simulink model "wptv1"  (R2024b)
settings: Solver=ode23tb  StartTime=0.0  StopTime=0.05  MaxStep=1e-7  RelTol=1e-3
libraries: spsSeriesRLCBranchLib x7, spsDiodeLib x5, spsMosfetLib x5, spsVoltageMeasurementLib x3, spsDCVoltageSourceLib x1, spsGroundLib x1, spsMutualInductanceLib x1, sps_lib x1
settings Model: Creator=barad  LastModifiedBy=barad

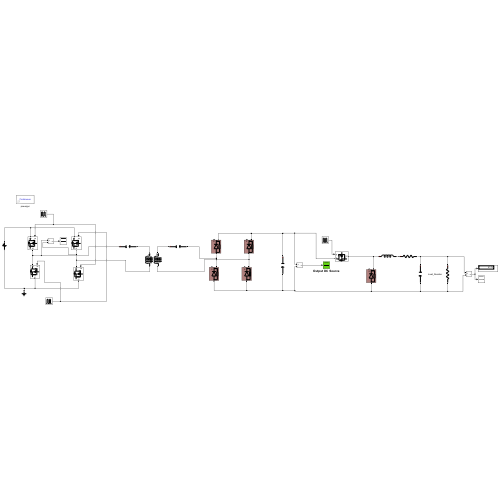
[thumbnail: Simulink's stored preview of the top-level diagram]
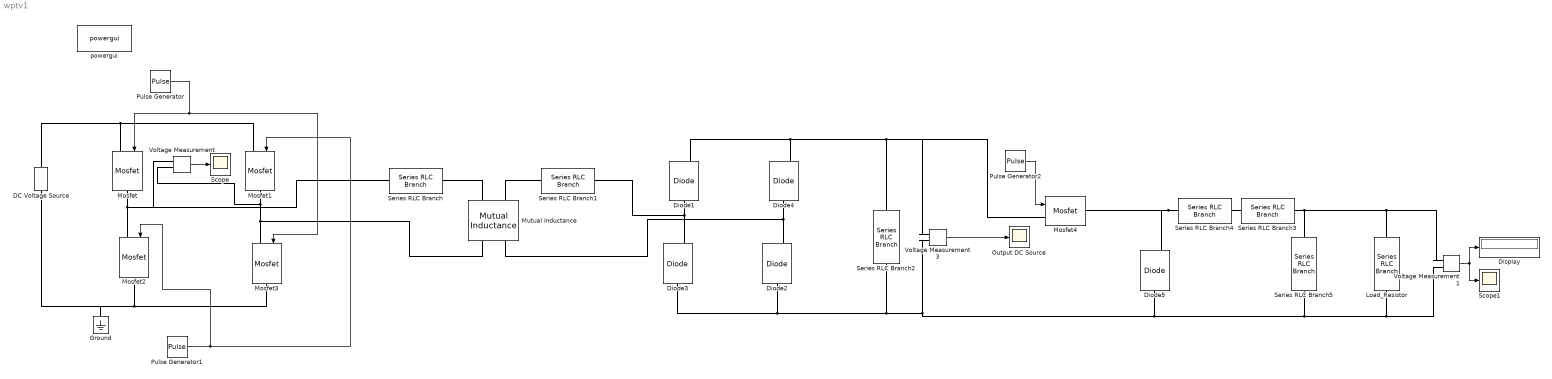
== system wptv1 ==
  DC Voltage Source : spsDCVoltageSourceLib/DC Voltage Source  Amplitude=24  Measurements=None
  Diode{1..5} (5 alike) : spsDiodeLib/Diode  Ron=0.001  Lon=0  Vf=0.8  IC=0  UseSnubber=0  Rs=500  Cs=250e-9  Measurements=on
  Display : Display
  Ground : spsGroundLib/Ground  LConnTagsString=a
  Load_Resistor : spsSeriesRLCBranchLib/Series RLC Branch  LConnTagsString=__new0  RConnTagsString=__new0  BranchType=R  Resistance=5.6  Inductance=100e-6  SetiL0=off  InitialCurrent=0  Capacitance=1e-6  Setx0=off  InitialVoltage=0  Measurements=None
  Mosfet{,1..3} (4 alike) : spsMosfetLib/Mosfet  Ron=0.007  Lon=0  Rd=0.01  Vfd=2.5  IC=0  Rs=1e5  Cs=150e-12  Measurements=off
  Mosfet4 : spsMosfetLib/Mosfet  Ron=0.007  Lon=0  Rd=0.01  Vfd=1.3  IC=0  Rs=1e5  Cs=inf  Measurements=off
  Mutual Inductance : spsMutualInductanceLib/Mutual Inductance  LConnTagsString=a|b  RConnTagsString=A|B  TypeOfMutual=Two or three windings with equal mutual terms  NumberOfWindings=3  SelfImpedance1=[0.3 15e-6]  SelfImpedance2=[0.3 15e-6]  ThreeWindings=off  SelfImpedance3=[ 1.1 1.1e-03]  MutualImpedance=[0 3e-6]  InductanceMatrix="[1.0 0.9  0.9 ;  0.9 1.0  0.9;  0.9 0.9 1.0 ] * 1e-3"  ResistanceMatrix="[1.0 0.9  0.9 ;  0.9 1.0  0.9;  0.9 0.9 1.0 ]"  Measurements=None
      settings: LibrarySourceBlock=sps_lib/Passives/Mutual Inductance
  Output DC Source : Scope
  Pulse Generator : DiscretePulseGenerator  PulseType=Time based  Period=1.176e-5  PulseWidth=50
  Pulse Generator1 : DiscretePulseGenerator  PulseType=Time based  Period=1.176e-5  PulseWidth=50  PhaseDelay=0.0000058824
  Pulse Generator2 : DiscretePulseGenerator  PulseType=Time based  Period=1/50000  PulseWidth=22
  Scope : Scope
  Scope1 : Scope
  Series RLC Branch : spsSeriesRLCBranchLib/Series RLC Branch  LConnTagsString=__new0  RConnTagsString=__new0  BranchType=C  Resistance=1  Inductance=1e-3  SetiL0=off  InitialCurrent=0  Capacitance=240e-9  Setx0=off  InitialVoltage=0  Measurements=None
  Series RLC Branch1 : spsSeriesRLCBranchLib/Series RLC Branch  LConnTagsString=__new0  RConnTagsString=__new0  BranchType=C  Resistance=1  Inductance=1e-3  SetiL0=off  InitialCurrent=0  Capacitance=240e-9  Setx0=off  InitialVoltage=0  Measurements=None
  Series RLC Branch2 : spsSeriesRLCBranchLib/Series RLC Branch  LConnTagsString=__new0  RConnTagsString=__new0  BranchType=C  Resistance=1  Inductance=1e-3  SetiL0=off  InitialCurrent=0  Capacitance=220e-6  Setx0=off  InitialVoltage=0  Measurements=None
  Series RLC Branch3 : spsSeriesRLCBranchLib/Series RLC Branch  LConnTagsString=__new0  RConnTagsString=__new0  BranchType=R  Resistance=0.02  Inductance=470e-6  SetiL0=off  InitialCurrent=0  Capacitance=1e-6  Setx0=off  InitialVoltage=0  Measurements=None
  Series RLC Branch4 : spsSeriesRLCBranchLib/Series RLC Branch  LConnTagsString=__new0  RConnTagsString=__new0  BranchType=L  Resistance=1  Inductance=470e-6  SetiL0=off  InitialCurrent=0  Capacitance=1e-6  Setx0=off  InitialVoltage=0  Measurements=None
  Series RLC Branch5 : spsSeriesRLCBranchLib/Series RLC Branch  LConnTagsString=__new0  RConnTagsString=__new0  BranchType=C  Resistance=1  Inductance=100e-6  SetiL0=off  InitialCurrent=0  Capacitance=100e-6  Setx0=off  InitialVoltage=0  Measurements=None
  Voltage Measurement : spsVoltageMeasurementLib/Voltage Measurement  PhasorSimulation=off  OutputType=Complex  PSBequivalent=0
  Voltage Measurement1 : spsVoltageMeasurementLib/Voltage Measurement  PhasorSimulation=off  OutputType=Complex  PSBequivalent=0
  Voltage Measurement3 : spsVoltageMeasurementLib/Voltage Measurement  PhasorSimulation=off  OutputType=Complex  PSBequivalent=0
  powergui : sps_lib/powergui  Priority=1  SimulationMode=Continuous  SampleTime=50e-6  frequency=60  Iterations=50  frequencyindice=0  Pbase=100e6  ErrMax=1e-4  UnitsV=kV  UnitsW=MW  buscounter=0  FunctionMessages=off  echomessages=off  EnableUseOfTLC=off  CurrentSourceSwitches=off  DisableSnubberDevices=off  DisableRonSwitches=off  DisableVfSwitches=off  DisplayEquations=off  AutomaticDiscreteSolvers=off  SolverType=Tustin/Backward Euler (TBE)  Interpol=off  ExternalGateDelay=off  methode=off  Ts=100  x0status=blocks  SPID=on  SwTol=0  HookPort=off  NonlinearTolerance=1e-4  nMaxIteration=100  ContinueOnMaxIteration=off  RestoreLinks=warning  ResistiveCurrentMeasurement=off  Frange=[0:2:500]  Ylog=off  Xlog=on  ShowGrid=off  save=off  variable=ZData  structure=0  ZoomFFT=off  StartTime=0.0  cycles=1  DisplayStyle=1  fundamental=60  FreqAxis=off  MaxFrequency=1000  frequencyindicesteady=1  RmsSteady=1  display=off
  wires:
  Pulse Generator/1 -> Mosfet3/1, Mosfet/1
  Pulse Generator1/1 -> Mosfet1/1, Mosfet2/1
  Voltage Measurement/1 -> Scope/1
  Voltage Measurement3/1 -> Output DC Source/1
  Pulse Generator2/1 -> Mosfet4/1
  Voltage Measurement1/1 -> Scope1/1, Display/1
  connections:
  Mosfet/LConn1 -- Mosfet1/LConn1 -- DC Voltage Source/RConn1
  Mosfet2/LConn1 -- Series RLC Branch/LConn1 -- Voltage Measurement/LConn1 -- Mosfet/RConn1
  Mosfet1/RConn1 -- Voltage Measurement/LConn2 -- Mutual Inductance/RConn1 -- Mosfet3/LConn1
  Mosfet3/RConn1 -- Ground/LConn1 -- DC Voltage Source/LConn1 -- Mosfet2/RConn1
  Mutual Inductance/LConn2 -- Series RLC Branch1/LConn1
  Mutual Inductance/LConn1 -- Series RLC Branch/RConn1
  Diode1/LConn1 -- Series RLC Branch1/RConn1 -- Diode3/RConn1
  Diode4/LConn1 -- Mutual Inductance/RConn2 -- Diode2/RConn1
  Load_Resistor/RConn1 -- Voltage Measurement1/LConn2 -- Diode5/LConn1 -- Voltage Measurement3/LConn2 -- Diode3/LConn1 -- Diode2/LConn1 -- Series RLC Branch2/RConn1 -- Series RLC Branch5/RConn1
  Diode1/RConn1 -- Series RLC Branch2/LConn1 -- Mosfet4/LConn1 -- Voltage Measurement3/LConn1 -- Diode4/RConn1
  Load_Resistor/LConn1 -- Voltage Measurement1/LConn1 -- Series RLC Branch3/RConn1 -- Series RLC Branch5/LConn1
  Series RLC Branch4/LConn1 -- Mosfet4/RConn1 -- Diode5/RConn1
  Series RLC Branch3/LConn1 -- Series RLC Branch4/RConn1
